simulink library "twist2pose"  (Simulink 7.9)
settings: Solver=ode45  StartTime=0.0  StopTime=10.0  RelTol=1e-3
settings Model: Creator=simena  LastModifiedBy=simena

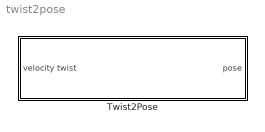
== system twist2pose ==
  Twist2Pose : Subsystem  mask{initial_pose=0, dt=0}
      mask prompts: initial_pose "Initial pose"; dt "Time sampling"
      mask help:
      | Compute the pose of the frame with the velocity given by the input
      |
      | Initial pose is a 6D vector with the initial position and euler angles (zyx) of the given frame

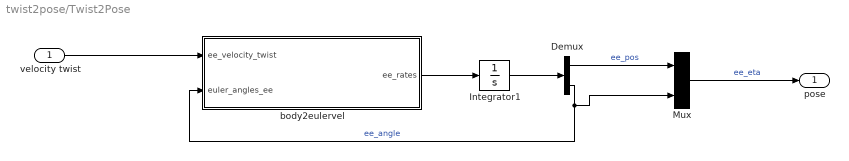
== system twist2pose/Twist2Pose ==
  velocity twist : Inport
  Demux : Demux  Outputs=2
  Integrator1 : Integrator  InitialCondition=initial_pose
  Mux : Mux  Inputs=2
  body2eulervel : MATLAB Function  TreatAsAtomicUnit=on
  pose : Outport
  wires:
  body2eulervel/1(ee_rates) -> Integrator1/1
  Integrator1/1 -> Demux/1
  Demux/2 -> body2eulervel/2(euler_angles_ee), Mux/2  "ee_angle"
  Demux/1 -> Mux/1  "ee_pos"
  velocity twist/1 -> body2eulervel/1(ee_velocity_twist)
  Mux/1 -> pose/1  "ee_eta"

== matlab function Twist2Pose/body2eulervel ==
  data: ee_velocity_twist input double size=6; ee_rates output double; euler_angles_ee input double size=3
function ee_rates = fcn(ee_velocity_twist, euler_angles_ee)                       
    %#codegen
       
    phi=euler_angles_ee(1);
    theta=euler_angles_ee(2);
    psi=euler_angles_ee(3);
    
    
    cphi = cos(phi);
    sphi = sin(phi);
    cth  = cos(theta);
    sth  = sin(theta);
 
    J1 = Rzyx(phi,theta,psi);
 
    if cth==0, error('J2 is singular for theta = +-90 degrees'); end
 
    J2 = [...
      1  sphi*sth/cth  cphi*sth/cth;
      0  cphi          -sphi;
      0  sphi/cth      cphi/cth ];
 
    J = [ J1  zeros(3,3);
      zeros(3,3) J2 ];
        
    ee_rates = zeros(6,1);
    ee_rates=J*ee_velocity_twist;
end



function R = Rzyx(phi,theta,psi)
    cphi = cos(phi);
    sphi = sin(phi);
    cth  = cos(theta);
    sth  = sin(theta);
    cpsi = cos(psi);
    spsi = sin(psi);

    R = [...
       cpsi*cth  -spsi*cphi+cpsi*sth*sphi  spsi*sphi+cpsi*cphi*sth
       spsi*cth  cpsi*cphi+sphi*sth*spsi   -cpsi*sphi+sth*spsi*cphi
       -sth      cth*sphi                  cth*cphi ];
end
